simulink model "sim_ROV_v0_R2018b"  (R2023a)
settings: Solver=ode4  StartTime=0.0  StopTime=sim_time  FixedStep=Ts  RelTol=1e-3
values from neighbouring files (symbols this model uses):
  B = rho*V*g*1.4    (= 168.9282)    [launcher_ROV_sim.m]    (also in lqr_design.m = [0.05581,         0,         0,         0,         0,       )
  D_linear = diag([D_u, D_v, D_w, D_p, D_q, D_r])    [launcher_ROV_sim.m]
  D_quadratic = diag([D_uu, D_vv, D_ww, D_pp, D_qq, D_rr])    [launcher_ROV_sim.m]
  force = lookup.Force_14V_Kgf    [launcher_ROV_sim.m]
  I = [I_xx   -I_xy   -I_xz ... (first row only)    [launcher_ROV_sim.m]
  Kq = [-14.0522937866 -0.000724361189881 7.36173354264e-14 -0.00802187271501 -1.59153029576 -0.00240388685004 -0.00102573418256 -14.0209983601 3.7395785387e-14 1.84702452338 0.00611607698573 0.00818162190067 ... (36 elements, 6x6)]    [lqr.mat]    (also in lqr_design.m = K(:,13:end))
  Kx = [30.0077125539 0.00159520383282 -9.18372190817e-14 0.0101724452135 3.59932945814 0.00293162043647 0.00170650423442 25.0803818094 -2.91671924306e-14 -3.06896094423 -0.00658141948351 -0.00836683203268 ... (72 elements, 6x12)]    [lqr.mat]    (also in lqr_design.m = K(:,1:12))
  m = 16.6    [launcher_ROV_sim.m]
  M_addedMass = [1.3169    0         0         0         0         0 ... (first row only)    [launcher_ROV_sim.m]
  M_rigidBody = [m        0        0        0          m*z_g     -m*y_g ... (first row only)    [launcher_ROV_sim.m]
  pwm = lookup.PWM    [launcher_ROV_sim.m]
  r_b = [x_b y_b z_b]'    [launcher_ROV_sim.m]
  r_g = [x_g y_g z_g]'    [launcher_ROV_sim.m]
  sim_time = 100    [launcher_ROV_sim.m]    (also in lqr_design.m)
  TCM = [ -0.7071   -0.7071    0.7071    0.7071    0         0         0         0 ... (first row only)    [launcher_ROV_sim.m]
  Ts = 0.01    [launcher_ROV_sim.m]    (also in lqr_design.m)
  W = m*g    (= 162.846)    [launcher_ROV_sim.m]
libraries: slpidlib x6, dspfdesign x6, simulink x2, aerolibnav x1, sharedtransform x1, aerolibanim x1
(part 2 of 2)

== system sim_ROV_v0_R2018b/Controller (LQR)/Test/Step ==
  Step : Step  Time=10  After=10  SampleTime=0
  Step1 : Step  Time=30  After=10  SampleTime=0
  Sum3 : Sum  Inputs=|+-
  step : Outport
  wires:
  Sum3/1 -> step/1
  Step1/1 -> Sum3/2
  Step/1 -> Sum3/1

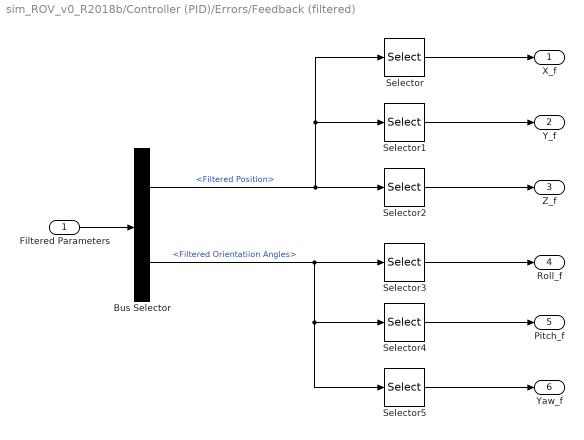
== system sim_ROV_v0_R2018b/Controller (PID)/Errors/Feedback (filtered) ==
  Filtered Parameters : Inport
  Bus Selector : BusSelector  OutputSignals=Filtered Position,Filtered Orientatiion Angles
  Selector : Selector  InputPortWidth=3  IndexOptions=Index vector (dialog)  Indices=1  OutputSizes=1
  Selector1 : Selector  InputPortWidth=3  IndexOptions=Index vector (dialog)  Indices=2  OutputSizes=1
  Selector2 : Selector  InputPortWidth=3  IndexOptions=Index vector (dialog)  Indices=3  OutputSizes=1
  Selector3 : Selector  InputPortWidth=3  IndexOptions=Index vector (dialog)  Indices=1  OutputSizes=1
  Selector4 : Selector  InputPortWidth=3  IndexOptions=Index vector (dialog)  Indices=2  OutputSizes=1
  Selector5 : Selector  InputPortWidth=3  IndexOptions=Index vector (dialog)  Indices=3  OutputSizes=1
  X_f : Outport  VectorParamsAs1DForOutWhenUnconnected=off
  Y_f : Outport  Port=2  VectorParamsAs1DForOutWhenUnconnected=off
  Z_f : Outport  Port=3  VectorParamsAs1DForOutWhenUnconnected=off
  Roll_f : Outport  Port=4  VectorParamsAs1DForOutWhenUnconnected=off
  Pitch_f : Outport  Port=5  VectorParamsAs1DForOutWhenUnconnected=off
  Yaw_f : Outport  Port=6  VectorParamsAs1DForOutWhenUnconnected=off
  wires:
  Filtered Parameters/1 -> Bus Selector/1
  Bus Selector/1 -> Selector/1, Selector1/1, Selector2/1  "<Filtered Position>"
  Bus Selector/2 -> Selector3/1, Selector4/1, Selector5/1  "<Filtered Orientatiion Angles>"
  Selector/1 -> X_f/1
  Selector1/1 -> Y_f/1
  Selector2/1 -> Z_f/1
  Selector3/1 -> Roll_f/1
  Selector4/1 -> Pitch_f/1
  Selector5/1 -> Yaw_f/1

== system sim_ROV_v0_R2018b/Controller (PID)/Errors/Reference Signals ==
  Reference : Inport
  Demux : Demux  Outputs=6
  X_ref : Outport  VectorParamsAs1DForOutWhenUnconnected=off
  Y_ref : Outport  Port=2  VectorParamsAs1DForOutWhenUnconnected=off
  Z_ref : Outport  Port=3  VectorParamsAs1DForOutWhenUnconnected=off
  Roll_ref : Outport  Port=4  VectorParamsAs1DForOutWhenUnconnected=off
  Pitch_ref : Outport  Port=5  VectorParamsAs1DForOutWhenUnconnected=off
  Yaw_ref : Outport  Port=6  VectorParamsAs1DForOutWhenUnconnected=off
  wires:
  Reference/1 -> Demux/1
  Demux/5 -> Pitch_ref/1
  Demux/4 -> Roll_ref/1
  Demux/3 -> Z_ref/1
  Demux/2 -> Y_ref/1
  Demux/6 -> Yaw_ref/1
  Demux/1 -> X_ref/1

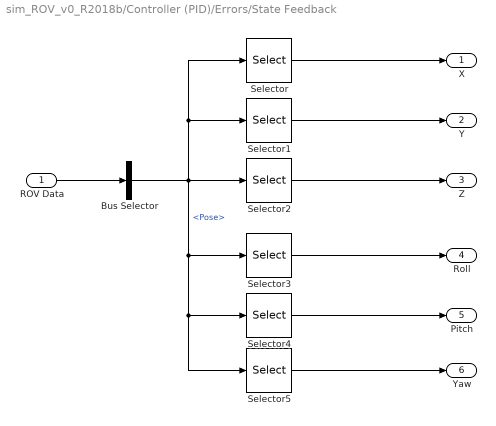
== system sim_ROV_v0_R2018b/Controller (PID)/Errors/State Feedback ==
  ROV Data : Inport
  Bus Selector : BusSelector  OutputSignals=Kinematics (Fixed).Pose
  Selector : Selector  InputPortWidth=6  IndexOptions=Index vector (dialog)  Indices=1  OutputSizes=1
  Selector1 : Selector  InputPortWidth=6  IndexOptions=Index vector (dialog)  Indices=2  OutputSizes=1
  Selector2 : Selector  InputPortWidth=6  IndexOptions=Index vector (dialog)  Indices=3  OutputSizes=1
  Selector3 : Selector  InputPortWidth=6  IndexOptions=Index vector (dialog)  Indices=4  OutputSizes=1
  Selector4 : Selector  InputPortWidth=6  IndexOptions=Index vector (dialog)  Indices=5  OutputSizes=1
  Selector5 : Selector  InputPortWidth=6  IndexOptions=Index vector (dialog)  Indices=6  OutputSizes=1
  X : Outport  VectorParamsAs1DForOutWhenUnconnected=off
  Y : Outport  Port=2  VectorParamsAs1DForOutWhenUnconnected=off
  Z : Outport  Port=3  VectorParamsAs1DForOutWhenUnconnected=off
  Roll : Outport  Port=4  VectorParamsAs1DForOutWhenUnconnected=off
  Pitch : Outport  Port=5  VectorParamsAs1DForOutWhenUnconnected=off
  Yaw : Outport  Port=6  VectorParamsAs1DForOutWhenUnconnected=off
  wires:
  ROV Data/1 -> Bus Selector/1
  Bus Selector/1 -> Selector5/1, Selector4/1, Selector3/1, Selector2/1, Selector1/1, Selector/1  "<Pose>"
  Selector4/1 -> Pitch/1
  Selector3/1 -> Roll/1
  Selector2/1 -> Z/1
  Selector1/1 -> Y/1
  Selector5/1 -> Yaw/1
  Selector/1 -> X/1

== system sim_ROV_v0_R2018b/Controller (PID)/Test/Chirp ==
  Chirp Signal : simulink/Sources/Chirp Signal  f1=0.005  T=sim_time  f2=1
  Gain : Gain  Gain=80
  chirp : Outport  VectorParamsAs1DForOutWhenUnconnected=off
  wires:
  Chirp Signal/1 -> Gain/1
  Gain/1 -> chirp/1

== system sim_ROV_v0_R2018b/Controller (PID)/Test/Impulse ==
  Derivative : Derivative
  Gain : Gain  Gain=0.001
  Step2 : Step  SampleTime=0
  impulse : Outport
  wires:
  Step2/1 -> Derivative/1
  Derivative/1 -> Gain/1
  Gain/1 -> impulse/1

== system sim_ROV_v0_R2018b/Controller (PID)/Test/Step ==
  Step : Step  Time=10  After=10  SampleTime=0
  Step1 : Step  Time=30  After=10  SampleTime=0
  Sum3 : Sum  Inputs=|+-
  step : Outport
  wires:
  Sum3/1 -> step/1
  Step1/1 -> Sum3/2
  Step/1 -> Sum3/1

== system sim_ROV_v0_R2018b/ROV (EVA)/Actuators Dynamics/Motors Transfer Functions ==
  pwm : Inport
  Demux : Demux  Outputs=8
  Mux : Mux  Inputs=8
  T200 Transfer Function {1..8} (8 alike) : TransferFcn  Numerator="[-107  8.358e04  3.989e04]"  Denominator="[1 152.9  3.036e04  2.93e06  1.157e06]"
  lbf : Outport  VectorParamsAs1DForOutWhenUnconnected=off
  wires:
  Demux/1 -> T200 Transfer Function 1/1
  T200 Transfer Function 4/1 -> Mux/4
  Demux/3 -> T200 Transfer Function 3/1
  Demux/8 -> T200 Transfer Function 8/1
  T200 Transfer Function 1/1 -> Mux/1
  T200 Transfer Function 5/1 -> Mux/5
  T200 Transfer Function 6/1 -> Mux/6
  Demux/2 -> T200 Transfer Function 2/1
  T200 Transfer Function 3/1 -> Mux/3
  Demux/5 -> T200 Transfer Function 5/1
  T200 Transfer Function 7/1 -> Mux/7
  Demux/6 -> T200 Transfer Function 6/1
  T200 Transfer Function 8/1 -> Mux/8
  T200 Transfer Function 2/1 -> Mux/2
  Demux/4 -> T200 Transfer Function 4/1
  Demux/7 -> T200 Transfer Function 7/1
  pwm/1 -> Demux/1
  Mux/1 -> lbf/1

== system sim_ROV_v0_R2018b/ROV (EVA)/ROV (non-linear)/Coriolis & Centripetal Forces ==
  Velocity : Inport
  Add : Sum
  Added Coriolis & Centripetal : MATLAB Function  TreatAsAtomicUnit=on
  Added Mass : Constant  Value=M_addedMass
  CoM : Constant  Value=r_g
  Inertia Tensor : Constant  Value=I
  Rigid Body Coriolis & Centripetal : MATLAB Function  TreatAsAtomicUnit=on
  Rigid Body Mass : Constant  Value=m
  F_C : Outport
  wires:
  Inertia Tensor/1 -> Rigid Body Coriolis & Centripetal/1(I)
  CoM/1 -> Rigid Body Coriolis & Centripetal/3(r_g)
  Rigid Body Mass/1 -> Rigid Body Coriolis & Centripetal/2(m)
  Added Mass/1 -> Added Coriolis & Centripetal/2(M_addedMass)
  Velocity/1 -> Added Coriolis & Centripetal/1(velocity), Rigid Body Coriolis & Centripetal/4(velocity)
  Added Coriolis & Centripetal/1(F_C_A) -> Add/2
  Add/1 -> F_C/1
  Rigid Body Coriolis & Centripetal/1(F_C_RB) -> Add/1

== system sim_ROV_v0_R2018b/ROV (EVA)/ROV (non-linear)/Damping Forces ==
  Velocity : Inport
  Abs : Abs  SaturateOnIntegerOverflow=off
  Linear Damping : Gain  Gain=D_linear  Multiplication=Matrix(K*u)
  Product : Product
  Quadratic Damping : Gain  Gain=D_quadratic  Multiplication=Matrix(K*u)
  Sum : Sum
  F_Drag : Outport
  wires:
  Product/1 -> Quadratic Damping/1
  Quadratic Damping/1 -> Sum/2
  Abs/1 -> Product/2
  Velocity/1 -> Abs/1, Product/1, Linear Damping/1
  Sum/1 -> F_Drag/1
  Linear Damping/1 -> Sum/1

== system sim_ROV_v0_R2018b/ROV (EVA)/ROV (non-linear)/Hydrostatics Forces ==
  Pose : Inport
  Attitude : Selector  InputPortWidth=6  IndexOptions=Index vector (dialog)  Indices=[4:6]  OutputSizes=1
  Buoyancy : Constant  Value=B
  CoB : Constant  Value=r_b
  CoM : Constant  Value=r_g
  Gravity Force : Constant  Value=W
  hydrostatics : MATLAB Function  TreatAsAtomicUnit=on
  F_g : Outport
  wires:
  Attitude/1 -> hydrostatics/1(attitude)
  hydrostatics/1(F_g) -> F_g/1
  Gravity Force/1 -> hydrostatics/2(W)
  Buoyancy/1 -> hydrostatics/3(B)
  CoM/1 -> hydrostatics/4(r_g)
  CoB/1 -> hydrostatics/5(r_b)
  Pose/1 -> Attitude/1

== system sim_ROV_v0_R2018b/ROV (EVA)/Rigid Body Dynamics/Coriolis & Centripetal Forces ==
  Velocity : Inport
  Add : Sum
  Added Coriolis & Centripetal : MATLAB Function  TreatAsAtomicUnit=on
  Added Mass : Constant  Value=M_addedMass
  CoM : Constant  Value=r_g
  Inertia Tensor : Constant  Value=I
  Rigid Body Coriolis & Centripetal : MATLAB Function  TreatAsAtomicUnit=on
  Rigid Body Mass : Constant  Value=m
  F_C : Outport
  wires:
  Inertia Tensor/1 -> Rigid Body Coriolis & Centripetal/1(I)
  CoM/1 -> Rigid Body Coriolis & Centripetal/3(r_g)
  Rigid Body Mass/1 -> Rigid Body Coriolis & Centripetal/2(m)
  Added Mass/1 -> Added Coriolis & Centripetal/2(M_addedMass)
  Velocity/1 -> Added Coriolis & Centripetal/1(velocity), Rigid Body Coriolis & Centripetal/4(velocity)
  Added Coriolis & Centripetal/1(F_C_A) -> Add/2
  Add/1 -> F_C/1
  Rigid Body Coriolis & Centripetal/1(F_C_RB) -> Add/1

== system sim_ROV_v0_R2018b/ROV (EVA)/Rigid Body Dynamics/Damping Forces ==
  Velocity : Inport
  Abs : Abs  SaturateOnIntegerOverflow=off
  Linear Damping : Gain  Gain=D_linear  Multiplication=Matrix(K*u)
  Product : Product
  Quadratic Damping : Gain  Gain=D_quadratic  Multiplication=Matrix(K*u)
  Sum : Sum
  F_Drag : Outport
  wires:
  Product/1 -> Quadratic Damping/1
  Quadratic Damping/1 -> Sum/2
  Abs/1 -> Product/2
  Velocity/1 -> Abs/1, Product/1, Linear Damping/1
  Sum/1 -> F_Drag/1
  Linear Damping/1 -> Sum/1

== system sim_ROV_v0_R2018b/ROV (EVA)/Rigid Body Dynamics/Hydrostatics Forces ==
  Pose : Inport
  Attitude : Selector  InputPortWidth=6  IndexOptions=Index vector (dialog)  Indices=[4:6]  OutputSizes=1
  Buoyancy : Constant  Value=B
  CoB : Constant  Value=r_b
  CoM : Constant  Value=r_g
  Gravity Force : Constant  Value=W
  hydrostatics : MATLAB Function  TreatAsAtomicUnit=on
  F_g : Outport
  wires:
  Attitude/1 -> hydrostatics/1(attitude)
  hydrostatics/1(F_g) -> F_g/1
  Gravity Force/1 -> hydrostatics/2(W)
  Buoyancy/1 -> hydrostatics/3(B)
  CoM/1 -> hydrostatics/4(r_g)
  CoB/1 -> hydrostatics/5(r_b)
  Pose/1 -> Attitude/1

== system sim_ROV_v0_R2018b/Visualization/3D Animation/3D Rotation ==
  "Roll, Pitch, Yaw" : Inport
  Points : Inport  Port=2
  Matrix Multiply : Product  Multiplication=Matrix(*)
  Rotation Angles to Direction Cosine Matrix : sharedtransform/Rotation Angles to Direction Cosine Matrix  rotationOrder=XYZ  aMode=aMode
  Transpose : Math  Operator=transpose  SignedPower=on
  Transformed : Outport  VectorParamsAs1DForOutWhenUnconnected=off
  wires:
  Rotation Angles to Direction Cosine Matrix/1 -> Transpose/1
  Transpose/1 -> Matrix Multiply/2
  Points/1 -> Matrix Multiply/1
  Matrix Multiply/1 -> Transformed/1
  "Roll, Pitch, Yaw"/1 -> Rotation Angles to Direction Cosine Matrix/1

== matlab function sim_ROV_v0_R2018b/ROV (EVA)/Rigid Body Dynamics/Hydrostatics Forces/hydrostatics ==
  data: attitude input; F_g output; W input; B input; r_g input; r_b input
function F_g = g(attitude,W,B,r_g,r_b)
%% Mapping
ph = attitude(1);
th = attitude(2);
ps = attitude(3);

x_g = r_g(1);
y_g = r_g(2);
z_g = r_g(3);

x_b = r_b(1);
y_b = r_b(2);
z_b = r_b(3);

%% Hydrostatics force
F_g = zeros(6,1);

F_g(1) = (W - B)*sin(th);
F_g(2) = -(W - B)*cos(th)*sin(ph);
F_g(3) = -(W - B)*cos(th)*cos(ph);
F_g(4) = -(y_g*W - y_b*B)*cos(th)*cos(ph) + (z_g*W - z_b*B)*cos(th)*sin(ph);
F_g(5) = (z_g*W - z_b*B)*sin(th) + (x_g*W - x_b*B)*cos(th)*cos(ph);
F_g(6) = -(x_g*W - x_b*B)*cos(th)*sin(ph) - (y_g*W - y_b*B)*sin(th);

end

== matlab function sim_ROV_v0_R2018b/ROV (EVA)/Rigid Body Dynamics/Coriolis & Centripetal Forces/Rigid Body Coriolis & Centripetal ==
  data: I input; m input; r_g input; velocity input; F_C_RB output
function F_C_RB = C_RB(I,m,r_g,velocity)

%% Mapping
% u = velocity(1);
% v = velocity(2);
% w = velocity(3);
% p = velocity(4);
% q = velocity(5);
% r = velocity(6);

%% Coriolis & Centripetal Matrix
% C11 = zeros(3);
% C12 = -m*skew(velocity(1:3)) - m*skew(velocity(4:6))*skew(r_g);
% C21 = -m*skew(velocity(1:3)) + m*skew(r_g)*skew(velocity(4:6));
% C22 = -skew(I*velocity(4:6));

C11 = m*skew(velocity(4:6));
C12 = -m*skew(velocity(4:6))*skew(r_g);
C21 = m*skew(r_g)*skew(velocity(4:6));
C22 = -skew(I*velocity(4:6));

C_RB = [C11 C12
        C21 C22];

%% Output
F_C_RB = C_RB*velocity;

end

%% Utilities
function S = skew(v)

if length(v) == 3

    S = [0       -v(3)     v(2)
         v(3)     0       -v(1)
        -v(2)     v(1)     0];

else

    ME = MException('MyComponent:inputError', ...
        'Input variable is not a 3 elements vector');
    throw(ME)
    
end

end

== matlab function sim_ROV_v0_R2018b/ROV (EVA)/Rigid Body Kinematics/kinematics ==
  data: eta_dot output; nu input; eta input
function eta_dot = kine(nu, eta)

%% Mapping
ph = eta(4,1);
th = eta(5,1);
ps = eta(6,1);

%% Matrices
% Rotation matrix (B -> I)
r11 = cos(ps)*cos(th);
r12 = -sin(ps)*cos(ph)+cos(ps)*sin(th)*sin(ph);
r13 = sin(ps)*sin(ph)+cos(ps)*cos(ph)*sin(th);

r21 = sin(ps)*cos(th);
r22 = cos(ps)*cos(ph)+sin(ph)*sin(th)*sin(ps);
r23 = -cos(ps)*sin(ph)+sin(th)*sin(ps)*cos(ph);

r31 = -sin(th);
r32 = cos(th)*sin(ph);
r33 = cos(th)*cos(ph);

R_bi = [r11 r12 r13
        r21 r22 r23
        r31 r32 r33];

% Matrix that relates the angular velocity vector with the derivatives of
% the Euler angles
T = [1     sin(ph)*tan(th)     cos(ph)*tan(th)
     0     cos(ph)            -sin(ph)
     0     sin(ph)/cos(th)     cos(ph)/cos(th)];

%% Output
Je = [R_bi       zeros(3)
      zeros(3)   T];

eta_dot = Je*nu;

end

== matlab function sim_ROV_v0_R2018b/ROV (EVA)/Rigid Body Dynamics/Coriolis & Centripetal Forces/Added Coriolis & Centripetal ==
  data: velocity input; F_C_A output; M_addedMass input
function F_C_A = C_A(velocity,M_addedMass)

%% Added Coriolis & Centripetal Matrix
a = M_addedMass*velocity;

C_A = [0         0         0         0        -a(3)      a(2)
       0         0         0         a(3)      0        -a(1)
       0         0         0        -a(2)      a(1)      0  
       0        -a(3)      a(2)      0        -a(6)      a(5)
       a(3)      0        -a(1)      a(6)      0        -a(4)
      -a(2)      a(1)      0        -a(5)      a(4)      0];

%% Output
F_C_A = C_A*velocity;

end

== matlab function sim_ROV_v0_R2018b/Visualization/3D Animation/MATLAB Function ==
  data: Position input; srf_in input
function Animation(Position, srf_in)

figure(1)

srf_in = srf_in + repmat([Position(1) Position(2) Position(3)],[16 1]);
plot3(srf_in(:,1),srf_in(:,2),srf_in(:,3),'b','linewidth',1.2);

xlim([-15 15]);
ylim([-15 15]);
zlim([-15 15]);

xlabel('$X[m]$','interpreter','latex','fontsize',15)
ylabel('$Y[m]$','interpreter','latex','fontsize',15)
zlabel('$Z[m]$','interpreter','latex','fontsize',15)

grid on

end

== matlab function sim_ROV_v0_R2018b/ROV (EVA)/Actuators Dynamics/Normalization ==
  data: u input; y output
function y = Normalize(u)
y = (u-1500)*150/400;
end

== matlab function sim_ROV_v0_R2018b/ROV (EVA)/ROV (non-linear)/Coriolis & Centripetal Forces/Added Coriolis & Centripetal ==
  data: velocity input; F_C_A output; M_addedMass input
function F_C_A = C_A(velocity,M_addedMass)

%% Added Coriolis & Centripetal Matrix
a = M_addedMass*velocity;

C_A = [0         0         0         0        -a(3)      a(2)
       0         0         0         a(3)      0        -a(1)
       0         0         0        -a(2)      a(1)      0  
       0        -a(3)      a(2)      0        -a(6)      a(5)
       a(3)      0        -a(1)      a(6)      0        -a(4)
      -a(2)      a(1)      0        -a(5)      a(4)      0];

%% Output
F_C_A = C_A*velocity;

end

== matlab function sim_ROV_v0_R2018b/ROV (EVA)/ROV (non-linear)/Coriolis & Centripetal Forces/Rigid Body Coriolis & Centripetal ==
  data: I input; m input; r_g input; velocity input; F_C_RB output
function F_C_RB = C_RB(I,m,r_g,velocity)

%% Mapping
% u = velocity(1);
% v = velocity(2);
% w = velocity(3);
% p = velocity(4);
% q = velocity(5);
% r = velocity(6);

%% Coriolis & Centripetal Matrix
% C11 = zeros(3);
% C12 = -m*skew(velocity(1:3)) - m*skew(velocity(4:6))*skew(r_g);
% C21 = -m*skew(velocity(1:3)) + m*skew(r_g)*skew(velocity(4:6));
% C22 = -skew(I*velocity(4:6));

C11 = m*skew(velocity(4:6));
C12 = -m*skew(velocity(4:6))*skew(r_g);
C21 = m*skew(r_g)*skew(velocity(4:6));
C22 = -skew(I*velocity(4:6));

C_RB = [C11 C12
        C21 C22];

%% Output
F_C_RB = C_RB*velocity;

end

%% Utilities
function S = skew(v)

if length(v) == 3

    S = [0       -v(3)     v(2)
         v(3)     0       -v(1)
        -v(2)     v(1)     0];

else

    ME = MException('MyComponent:inputError', ...
        'Input variable is not a 3 elements vector');
    throw(ME)
    
end

end

== matlab function sim_ROV_v0_R2018b/ROV (EVA)/ROV (non-linear)/Hydrostatics Forces/hydrostatics ==
  data: attitude input; F_g output; W input; B input; r_g input; r_b input
function F_g = g(attitude,W,B,r_g,r_b)
%% Mapping
ph = attitude(1);
th = attitude(2);
ps = attitude(3);

x_g = r_g(1);
y_g = r_g(2);
z_g = r_g(3);

x_b = r_b(1);
y_b = r_b(2);
z_b = r_b(3);

%% Hydrostatics force
F_g = zeros(6,1);

F_g(1) = (W - B)*sin(th);
F_g(2) = -(W - B)*cos(th)*sin(ph);
F_g(3) = -(W - B)*cos(th)*cos(ph);
F_g(4) = -(y_g*W - y_b*B)*cos(th)*cos(ph) + (z_g*W - z_b*B)*cos(th)*sin(ph);
F_g(5) = (z_g*W - z_b*B)*sin(th) + (x_g*W - x_b*B)*cos(th)*cos(ph);
F_g(6) = -(x_g*W - x_b*B)*cos(th)*sin(ph) - (y_g*W - y_b*B)*sin(th);

end

== matlab function sim_ROV_v0_R2018b/ROV (EVA)/ROV (non-linear)/kinematics ==
  data: eta_dot output; nu input; eta input
function eta_dot = kine(nu, eta)

%% Mapping
ph = eta(4,1);
th = eta(5,1);
ps = eta(6,1);

%% Matrices
% Rotation matrix (B -> I)
r11 = cos(ps)*cos(th);
r12 = -sin(ps)*cos(ph)+cos(ps)*sin(th)*sin(ph);
r13 = sin(ps)*sin(ph)+cos(ps)*cos(ph)*sin(th);

r21 = sin(ps)*cos(th);
r22 = cos(ps)*cos(ph)+sin(ph)*sin(th)*sin(ps);
r23 = -cos(ps)*sin(ph)+sin(th)*sin(ps)*cos(ph);

r31 = -sin(th);
r32 = cos(th)*sin(ph);
r33 = cos(th)*cos(ph);

R_bi = [r11 r12 r13
        r21 r22 r23
        r31 r32 r33];

% Matrix that relates the angular velocity vector with the derivatives of
% the Euler angles
T = [1     sin(ph)*tan(th)     cos(ph)*tan(th)
     0     cos(ph)            -sin(ph)
     0     sin(ph)/cos(th)     cos(ph)/cos(th)];

%% Output
Je = [R_bi       zeros(3)
      zeros(3)   T];

eta_dot = Je*nu;

end
